simulink model "untitled"  (R2014a)
settings: Solver=ode45  StartTime=0.0  StopTime=10.0  RelTol=1e-3
settings Model: Creator=HamOs  LastModifiedBy=Hamlet

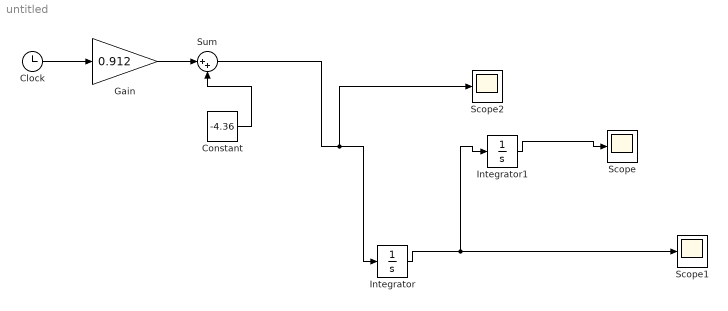
== system untitled ==
  Clock : Clock
  Constant : Constant  Value=-4.36
  Gain : Gain  Gain=0.912
  Integrator : Integrator  InitialCondition=6  LowerSaturationLimit=0
  Integrator1 : Integrator  InitialCondition=12  UpperSaturationLimit=10  LowerSaturationLimit=0
  Scope : Scope
      settings: ShowLegends=on
  Scope1 : Scope
      settings: TimeRange=10  YMax=10
  Scope2 : Scope
      settings: TimeRange=10  SaveName=ScopeData2
  Sum : Sum  Inputs=|++
  wires:
  Clock/1 -> Gain/1
  Gain/1 -> Sum/1
  Integrator/1 -> Integrator1/1, Scope1/1
  Integrator1/1 -> Scope/1
  Constant/1 -> Sum/2
  Sum/1 -> Scope2/1, Integrator/1
